simulink model "aufgabe1_linear_anfangsbedingung2"  (R2023b)
settings: Solver=FixedStepAuto  StartTime=0.0  StopTime=10.0  FixedStep=0.001  RelTol=1e-3
settings Model: Creator=serkan  LastModifiedBy=serkan

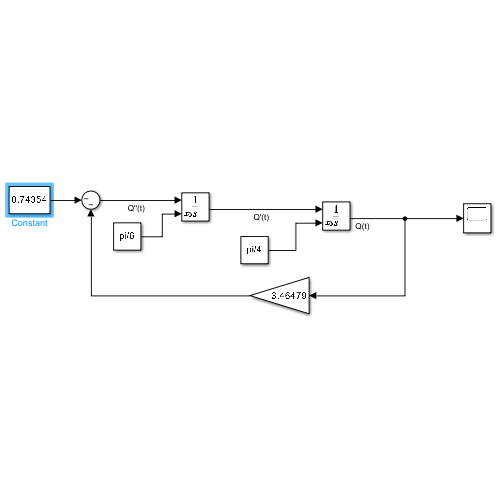
[thumbnail: Simulink's stored preview of the top-level diagram]
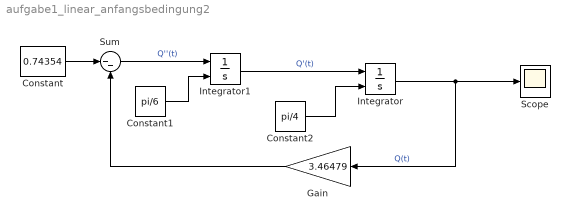
== system aufgabe1_linear_anfangsbedingung2 ==
  Constant : Constant  Value=0.74354
  Constant1 : Constant  Value=pi/6
  Constant2 : Constant  Value=pi/4
  Gain : Gain  Gain=3.46479
  Integrator : Integrator  InitialConditionSource=external  InitialCondition=pi/6
  Integrator1 : Integrator  InitialConditionSource=external
  Scope : Scope
  Sum : Sum  Inputs=|--
  wires:
  Constant/1 -> Sum/1
  Gain/1 -> Sum/2
  Integrator/1 -> Gain/1, Scope/1  "Q(t)"
  Integrator1/1 -> Integrator/1  "Q'(t)"
  Sum/1 -> Integrator1/1  "Q''(t)"
  Constant1/1 -> Integrator1/2
  Constant2/1 -> Integrator/2
